simulink model "offline_snac_SITL"  (R2024a)
settings: Solver=FixedStepDiscrete  StartTime=0.0  StopTime=50  FixedStep=0.001  RelTol=1e-3  EnableMultiTasking=on
undefined symbols (not defined in the file or in its folder): DiscIntNeverNeededParam
libraries: simulink x6, px4uORBlib x3, sharedtransform x1, px4lib x1
settings Model: ExtModeTrigDuration=10  Creator=re606359  LastModifiedBy=engelhardt
settings SolverCC: PositivePriorityOrder=on
settings OptimizationCC: EnhancedBackFolding=on  PassReuseOutputArgsAs=Individual arguments  ZeroExternalMemoryAtStartup=off  ZeroInternalMemoryAtStartup=off  MaxStackSize=64  OptimizeBlockOrder=speed  DifferentSizesBufferReuse=on  OptimizationCustomize=off  EfficientTunableParamExpr=on
settings DebuggingCC: ParameterTunabilityLossMsg=error
settings HardwareCC: ProdBitPerPointer=32  ProdBitPerSizeT=32  ProdBitPerPtrDiffT=32  ProdLargestAtomicInteger=Long  ProdLargestAtomicFloat=Double  ProdWordSize=32  ProdLongLongMode=on  ProdHWDeviceType=ARM Compatible->ARM Cortex
settings SFSimCC: MATLABDynamicMemAlloc=off  SimTargetLang=C++
settings RTWCC: Description=Embedded Coder  SystemTargetFile=ert.tlc  HardwareBoard=PX4 Host Target  TLCOptions="-aInlineSetEventsForThisBaseRateFcn=TLC_FALSE -aSuppressMultiTaskScheduler=TLC_FALSE  -aRateBasedStepFcn=0"  TemplateMakefile=ert_default_tmf  Toolchain=GNU Tools for PX4 Autopilots  PortableWordSizes=on  TargetLang=C++  GPUComputeCapability=3.5
settings CodeAppCC: ForceParamTrailComments=on  IgnoreCustomStorageClasses=off  OperatorAnnotations=on  SimulinkDataObjDesc=on  SFDataObjDesc=on  InsertBlockDesc=on
settings ERTTargetCC: SupportContinuousTime=on  ExtModeTransport=2  ExtModeStaticAlloc=on  ExtModeMexFile=ext_xcp  ExtModeIntrfLevel=Level2 - Open

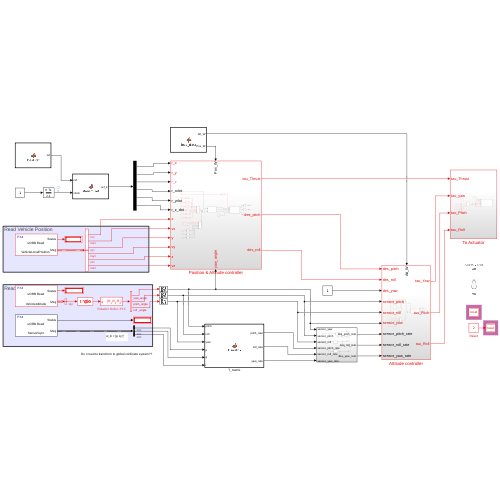
[thumbnail: Simulink's stored preview of the top-level diagram]
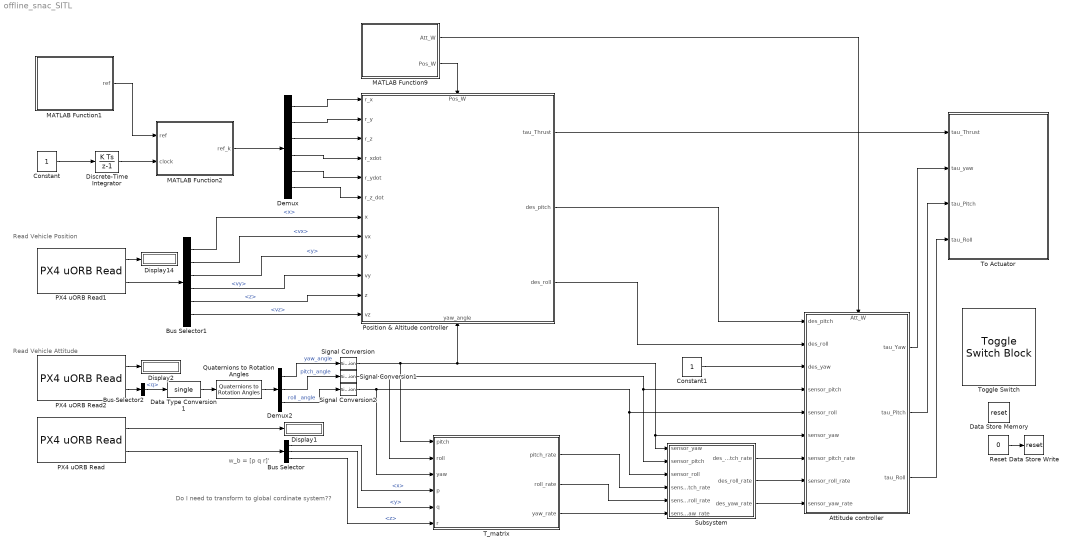
== system offline_snac_SITL ==
  note: w_b = [p q r]'
  note: Do I need to transform to global cordinate system??
  note: Read Vehicle Position
  note: Read Vehicle Attitude
  Attitude controller : Subsystem
      settings: PortSchema="{\"entries\":[{\"content\":{\"sides\":[{\"content\":{\"connectorIds\":[\"In1\",\"In2\",\"In3\",\"In4\",\"In5\",\"In6\",\"In7\",\"In8\",\"In9\"]},\"type\":\"ConnectorPlacement.EquallySpacedRectSide\",\"uuid\":\"fae962e8-eaa0-4300-aebb-2542e8dc0b9d\"},{\"content\":{\"connectorIds\":[\"Out1\",\"Out2\",\"Out3\"],\"side\":\"RIGHT\"},\"type\":\"ConnectorPlacement.EquallySpacedRectSide\",\"uuid\":\"2ab64516-4178-4987-b105-e2b60ebc653b\"},{\"content\":{\"connectorIds\":[\"In10\"],\"side\":\"TOP\"},\"type\":\"ConnectorPlacement.EquallySpacedRectSide\",\"uuid\":\"8c218eee-bea7-4b7a-ab96-9bd58138bc2f\"},{\"content\":{\"side\":\"BOTTOM\"},\"type\":\"ConnectorPlacement.EquallySpacedRectSide\",\"uuid\":\"12c5faa8-5812-413f-bdcf-aa5ffbd59e54\"}]},\"type\":\"ConnectorPlacement.EquallySpacedConnector\",\"uuid\":\"49b20a1e-3c6c-4df6-a9b5-cb8878061c64\"}],\"packageUris\":[\"http://schema.mathworks.com/mf0/Connector/R2020b\"],\"version\":\"1.0\"}"
  Bus Selector : BusSelector  OutputSignals=x,y,z
  Bus Selector1 : BusSelector  OutputSignals=x,vx,y,vy,z,vz
  Bus Selector2 : BusSelector  OutputSignals=q
  Constant : Constant  OutDataTypeStr=single
  Constant1 : Constant  OutDataTypeStr=single
  Data Store Write : DataStoreWrite  DataStoreName=reset  IndexOptions=Index vector (dialog)  Indices=1  OutputSizes=1
  Data Store Memory : DataStoreMemory  DataStoreName=reset  ReadBeforeWriteMsg=warning  WriteAfterWriteMsg=warning  WriteAfterReadMsg=warning  ShowAdditionalParam=off  OutDataTypeStr=boolean
  Data Type Conversion1 : DataTypeConversion  OutDataTypeStr=single  SaturateOnIntegerOverflow=off  RndMeth=Floor
  Demux : Demux  Outputs=6
  Demux2 : Demux  Outputs=3
  Discrete-Time Integrator : DiscreteIntegrator  SampleTime=-1  ICPrevOutput=DiscIntNeverNeededParam  ICPrevScaledInput=DiscIntNeverNeededParam
  Display1 : Display
  Display14 : Display
  Display2 : Display
  MATLAB Function1 : MATLAB Function  TreatAsAtomicUnit=on
  MATLAB Function2 : MATLAB Function  TreatAsAtomicUnit=on
  MATLAB Function9 : MATLAB Function  TreatAsAtomicUnit=on
  PX4 uORB Read : px4uORBlib/PX4 uORB Read  uORBTopic=SensorGyro  selectInstance=SensorGyro  SampleTime=-1  BlockingMode=off  BlockTimeout=1e-3
  PX4 uORB Read1 : px4uORBlib/PX4 uORB Read  uORBTopic=VehicleLocalPosition  selectInstance=vehicle_local_position  SampleTime=-1  BlockingMode=off  BlockTimeout=1e-3
  PX4 uORB Read2 : px4uORBlib/PX4 uORB Read  uORBTopic=VehicleAttitude  selectInstance=vehicle_attitude  SampleTime=-1  BlockingMode=off  BlockTimeout=1e-3
  Position & Altitude controller : Subsystem
      settings: PortSchema="{\"entries\":[{\"content\":{\"sides\":[{\"content\":{\"connectorIds\":[\"In1\",\"In2\",\"In3\",\"In4\",\"In5\",\"In6\",\"In7\",\"In8\",\"In9\",\"In10\",\"In11\",\"In12\"]},\"type\":\"ConnectorPlacement.EquallySpacedRectSide\",\"uuid\":\"96eb1e1d-33f8-43b2-aca1-3a2ea17c97d3\"},{\"content\":{\"connectorIds\":[\"Out1\",\"Out2\",\"Out3\"],\"side\":\"RIGHT\"},\"type\":\"ConnectorPlacement.EquallySpacedRectSide\",\"uuid\":\"68c63f59-0b7f-4dee-beff-edcde1fd911b\"},{\"content\":{\"connectorIds\":[\"In13\"],\"side\":\"TOP\"},\"type\":\"ConnectorPlacement.EquallySpacedRectSide\",\"uuid\":\"695c40b8-e625-4f49-aae8-ed972e1604cc\"},{\"content\":{\"connectorIds\":[\"In14\"],\"side\":\"BOTTOM\"},\"type\":\"ConnectorPlacement.EquallySpacedRectSide\",\"uuid\":\"eed3d45c-6018-4bc3-85c5-6c8aa0ab95cc\"}]},\"type\":\"ConnectorPlacement.EquallySpacedConnector\",\"uuid\":\"b4b28bb8-7674-4138-b24e-55baa1b4cc5c\"}],\"packageUris\":[\"http://schema.mathworks.com/mf0/Connector/R2020b\"],\"version\":\"1.0\"}"
  Quaternions to Rotation Angles : sharedtransform/Quaternions to Rotation Angles  rotationOrder=ZYX  aMode=aMode
  Reset : Constant  Value=0  OutDataTypeStr=boolean  SampleTime=-1
      settings: OpenFcn=|
      | if strcmp('0',get_param(gcb, 'Value'))                        set_param(gcb, 'Value', '1');
      | else
      |             set_param(gcb, 'Value', '0');
      | end
  Signal Conversion : SignalConversion  OverrideOpt=off
  Signal Conversion1 : SignalConversion  OverrideOpt=off
  Signal Conversion2 : SignalConversion  OverrideOpt=off
  Subsystem : Subsystem
  T_matrix : MATLAB Function  TreatAsAtomicUnit=on
  To Actuator : Subsystem
  Toggle Switch : ToggleSwitchBlock
      settings: Values={{'Off', 'On'}, [0 1]}
  wires:
  Bus Selector1/5 -> Position & Altitude controller/11(z)  "<z>"
  Demux2/1 -> Signal Conversion/1  "yaw_angle"
  PX4 uORB Read2/2 -> Bus Selector2/1
  Position & Altitude controller/1(tau_Thrust) -> To Actuator/1(tau_Thrust)
  Attitude controller/2(tau_Pitch) -> To Actuator/3(tau_Pitch)
  Demux2/3 -> Signal Conversion2/1  "roll _angle"
  Position & Altitude controller/3(des_roll) -> Attitude controller/2(des_roll)
  Signal Conversion/1 -> T_matrix/1(pitch), Attitude controller/6(sensor_yaw), Subsystem/1(sensor_yaw), Position & Altitude controller/14(yaw_angle)
  Bus Selector1/3 -> Position & Altitude controller/9(y)  "<y>"
  Attitude controller/1(tau_Yaw) -> To Actuator/2(tau_yaw)
  Quaternions to Rotation Angles/1 -> Demux2/1
  Bus Selector1/6 -> Position & Altitude controller/12(vz)  "<vz>"
  PX4 uORB Read2/1 -> Display2/1
  Position & Altitude controller/2(des_pitch) -> Attitude controller/1(des_pitch)
  Attitude controller/3(tau_Roll) -> To Actuator/4(tau_Roll)
  Demux2/2 -> Signal Conversion1/1  "pitch_angle"
  PX4 uORB Read1/1 -> Display14/1
  PX4 uORB Read1/2 -> Bus Selector1/1
  Signal Conversion1/1 -> T_matrix/2(roll), Subsystem/2(sensor_pitch), Attitude controller/4(sensor_pitch)
  Signal Conversion2/1 -> T_matrix/3(yaw), Subsystem/3(sensor_roll), Attitude controller/5("sensor_roll ")
  Bus Selector1/1 -> Position & Altitude controller/7(x)  "<x>"
  Bus Selector1/4 -> Position & Altitude controller/10(vy)  "<vy>"
  Bus Selector1/2 -> Position & Altitude controller/8(vx)  "<vx>"
  Reset/1 -> Data Store Write/1
  Bus Selector2/1 -> Data Type Conversion1/1  "<q>"
  Data Type Conversion1/1 -> Quaternions to Rotation Angles/1
  MATLAB Function9/2(Pos_W) -> Position & Altitude controller/13(Pos_W)
  MATLAB Function9/1(Att_W) -> Attitude controller/10(Att_W)
  PX4 uORB Read/1 -> Display1/1
  PX4 uORB Read/2 -> Bus Selector/1
  T_matrix/1(pitch_rate) -> Subsystem/4(sensor_pitch_rate)
  T_matrix/3(yaw_rate) -> Subsystem/6(sensor_yaw_rate)
  Bus Selector/1 -> T_matrix/4(p)  "<x>"
  Bus Selector/2 -> T_matrix/5(q)  "<y>"
  Bus Selector/3 -> T_matrix/6(r)  "<z>"
  T_matrix/2(roll_rate) -> Subsystem/5(sensor_roll_rate)
  MATLAB Function1/1(ref) -> MATLAB Function2/1(ref)
  Discrete-Time Integrator/1 -> MATLAB Function2/2(clock)
  Constant/1 -> Discrete-Time Integrator/1
  MATLAB Function2/1(ref_k) -> Demux/1
  Demux/1 -> Position & Altitude controller/1(r_x)
  Demux/2 -> Position & Altitude controller/2(r_y)
  Demux/3 -> Position & Altitude controller/3(r_z)
  Demux/4 -> Position & Altitude controller/4(r_xdot)
  Demux/5 -> Position & Altitude controller/5(r_ydot)
  Demux/6 -> Position & Altitude controller/6(r_z_dot)
  Subsystem/1(des_pitch_rate) -> Attitude controller/7(sensor_pitch_rate)
  Subsystem/2(des_roll_rate) -> Attitude controller/8(sensor_roll_rate)
  Subsystem/3(des_yaw_rate) -> Attitude controller/9(sensor_yaw_rate)
  Constant1/1 -> Attitude controller/3(des_yaw)

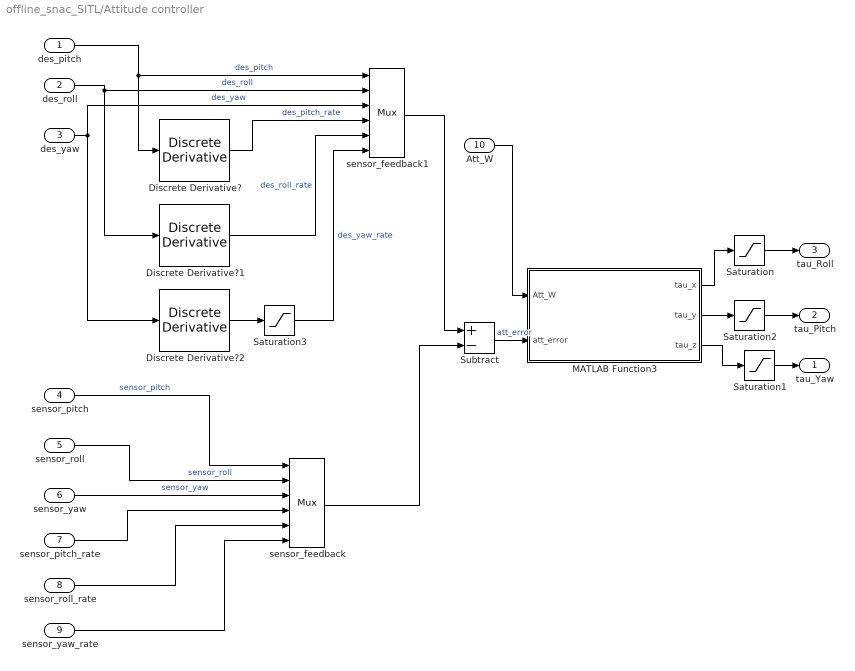
== system offline_snac_SITL/Attitude controller ==
  des_pitch : Inport  OutDataTypeStr=single
  des_roll : Inport  Port=2  OutDataTypeStr=single
  des_yaw : Inport  Port=3  OutDataTypeStr=single
  sensor_pitch : Inport  Port=4
  "sensor_roll " : Inport  Port=5
  sensor_yaw : Inport  Port=6
  sensor_pitch_rate : Inport  Port=7
  sensor_roll_rate : Inport  Port=8
  sensor_yaw_rate : Inport  Port=9
  Att_W : Inport  Port=10
  Discrete Derivative? : simulink/Discrete/Discrete Derivative  gainval=1.0  ICPrevScaledInput=0.0  OutMin=[]  OutMax=[]  OutDataTypeStr=single  OutputDataTypeScalingMode=single  OutDataType=fixdt(1, 16)  OutScaling=2^-10  DoSatur=off
  Discrete Derivative?1 : simulink/Discrete/Discrete Derivative  gainval=1.0  ICPrevScaledInput=0.0  OutMin=[]  OutMax=[]  OutDataTypeStr=single  OutputDataTypeScalingMode=single  OutDataType=fixdt(1, 16)  OutScaling=2^-10  DoSatur=off
  Discrete Derivative?2 : simulink/Discrete/Discrete Derivative  gainval=1.0  ICPrevScaledInput=0.0  OutMin=[]  OutMax=[]  OutDataTypeStr=single  OutputDataTypeScalingMode=single  OutDataType=fixdt(1, 16)  OutScaling=2^-10  DoSatur=off
  MATLAB Function3 : MATLAB Function  TreatAsAtomicUnit=on
  Saturation : Saturate  UpperLimit=8  LowerLimit=-8
  Saturation1 : Saturate  UpperLimit=3  LowerLimit=-3
  Saturation2 : Saturate  UpperLimit=8  LowerLimit=-8
  Saturation3 : Saturate  UpperLimit=1  LowerLimit=-1
  Subtract : Sum  Inputs=+-
  sensor_feedback : Mux  Inputs=6
  sensor_feedback1 : Mux  Inputs=6
  tau_Yaw : Outport
  tau_Pitch : Outport  Port=2
  tau_Roll : Outport  Port=3
  wires:
  sensor_pitch/1 -> sensor_feedback/1  "sensor_pitch"
  "sensor_roll "/1 -> sensor_feedback/2  "sensor_roll"
  sensor_yaw/1 -> sensor_feedback/3  "sensor_yaw"
  sensor_pitch_rate/1 -> sensor_feedback/4
  sensor_roll_rate/1 -> sensor_feedback/5
  sensor_yaw_rate/1 -> sensor_feedback/6
  sensor_feedback/1 -> Subtract/2
  Att_W/1 -> MATLAB Function3/1(Att_W)
  Subtract/1 -> MATLAB Function3/2(att_error)  "att_error"
  des_pitch/1 -> Discrete Derivative?/1, sensor_feedback1/1  "des_pitch"
  des_roll/1 -> Discrete Derivative?1/1, sensor_feedback1/2  "des_roll"
  des_yaw/1 -> Discrete Derivative?2/1, sensor_feedback1/3  "des_yaw"
  Saturation3/1 -> sensor_feedback1/6  "des_yaw_rate"
  Discrete Derivative?1/1 -> sensor_feedback1/5  "des_roll_rate"
  Discrete Derivative?/1 -> sensor_feedback1/4  "des_pitch_rate"
  sensor_feedback1/1 -> Subtract/1
  MATLAB Function3/1(tau_x) -> Saturation/1
  Saturation/1 -> tau_Roll/1
  Saturation2/1 -> tau_Pitch/1
  MATLAB Function3/2(tau_y) -> Saturation2/1
  Saturation1/1 -> tau_Yaw/1
  MATLAB Function3/3(tau_z) -> Saturation1/1
  Discrete Derivative?2/1 -> Saturation3/1

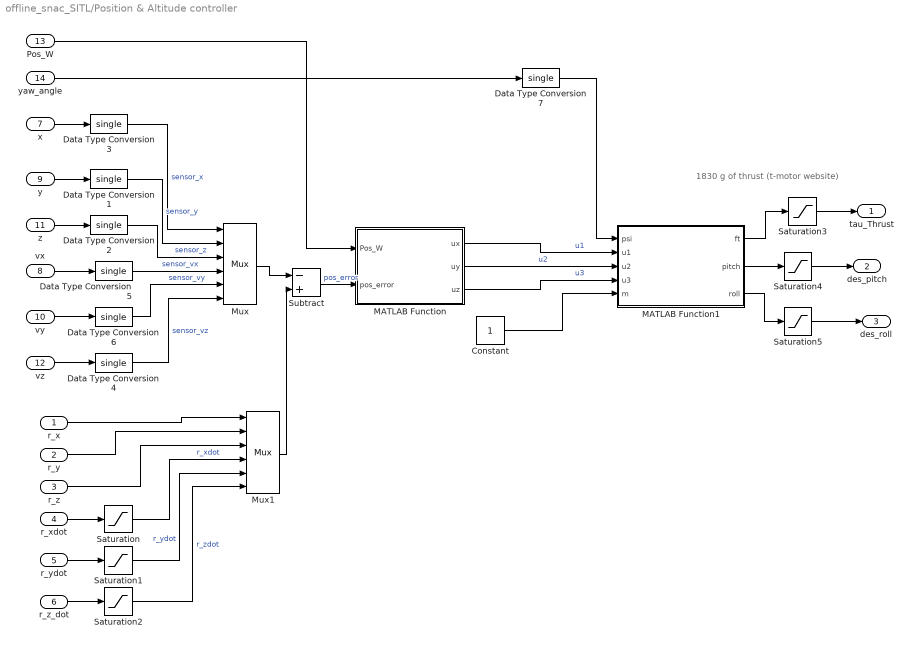
== system offline_snac_SITL/Position & Altitude controller ==
  note: 1830 g of thrust (t-motor website)
  r_x : Inport
  r_y : Inport  Port=2
  r_z : Inport  Port=3
  r_xdot : Inport  Port=4
  r_ydot : Inport  Port=5
  r_z_dot : Inport  Port=6
  x : Inport  Port=7
  vx : Inport  Port=8
  y : Inport  Port=9
  vy : Inport  Port=10
  z : Inport  Port=11
  vz : Inport  Port=12
  Pos_W : Inport  Port=13
  yaw_angle : Inport  Port=14
  Constant : Constant  OutDataTypeStr=single
  Data Type Conversion{1..7} (7 alike) : DataTypeConversion  OutDataTypeStr=single  SaturateOnIntegerOverflow=off  RndMeth=Floor
  MATLAB Function : MATLAB Function  TreatAsAtomicUnit=on
  MATLAB Function1 : MATLAB Function  TreatAsAtomicUnit=on
  Mux : Mux  Inputs=6
  Mux1 : Mux  Inputs=6
  Saturation : Saturate  UpperLimit=15  LowerLimit=-15
  Saturation1 : Saturate  UpperLimit=15  LowerLimit=-15
  Saturation2 : Saturate  UpperLimit=15  LowerLimit=-15
  Saturation3 : Saturate  UpperLimit=72  LowerLimit=0
  Saturation4 : Saturate  UpperLimit=.79  LowerLimit=-.79
  Saturation5 : Saturate  UpperLimit=.79  LowerLimit=-.79
  Subtract : Sum  Inputs=-+
  tau_Thrust : Outport  OutDataTypeStr=single
  des_pitch : Outport  Port=2
  des_roll : Outport  Port=3
  wires:
  z/1 -> Data Type Conversion2/1
  x/1 -> Data Type Conversion3/1
  y/1 -> Data Type Conversion1/1
  vz/1 -> Data Type Conversion4/1
  vx/1 -> Data Type Conversion5/1
  vy/1 -> Data Type Conversion6/1
  Pos_W/1 -> MATLAB Function/1(Pos_W)
  Data Type Conversion3/1 -> Mux/1  "sensor_x"
  Data Type Conversion1/1 -> Mux/2  "sensor_y"
  Data Type Conversion2/1 -> Mux/3  "sensor_z"
  Data Type Conversion5/1 -> Mux/4  "sensor_vx"
  Data Type Conversion6/1 -> Mux/5  "sensor_vy"
  Data Type Conversion4/1 -> Mux/6  "sensor_vz"
  Mux/1 -> Subtract/1
  Mux1/1 -> Subtract/2
  r_x/1 -> Mux1/1
  r_y/1 -> Mux1/2
  r_z/1 -> Mux1/3
  Subtract/1 -> MATLAB Function/2(pos_error)  "pos_error"
  Constant/1 -> MATLAB Function1/5(m)
  MATLAB Function/1(ux) -> MATLAB Function1/2(u1)  "u1"
  yaw_angle/1 -> Data Type Conversion7/1
  MATLAB Function/2(uy) -> MATLAB Function1/3(u2)  "u2"
  MATLAB Function/3(uz) -> MATLAB Function1/4(u3)  "u3"
  Data Type Conversion7/1 -> MATLAB Function1/1(psi)
  r_ydot/1 -> Saturation1/1
  r_z_dot/1 -> Saturation2/1
  r_xdot/1 -> Saturation/1
  Saturation/1 -> Mux1/4  "r_xdot"
  Saturation1/1 -> Mux1/5  "r_ydot"
  Saturation2/1 -> Mux1/6  "r_zdot"
  Saturation3/1 -> tau_Thrust/1
  MATLAB Function1/1(ft) -> Saturation3/1
  MATLAB Function1/2(pitch) -> Saturation4/1
  Saturation4/1 -> des_pitch/1
  Saturation5/1 -> des_roll/1
  MATLAB Function1/3(roll) -> Saturation5/1

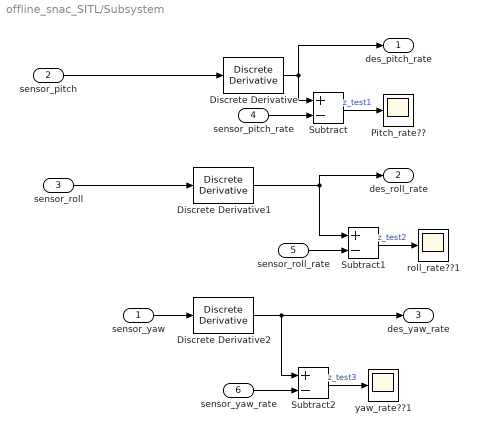
== system offline_snac_SITL/Subsystem ==
  sensor_yaw : Inport
  sensor_pitch : Inport  Port=2
  sensor_roll : Inport  Port=3
  sensor_pitch_rate : Inport  Port=4
  sensor_roll_rate : Inport  Port=5
  sensor_yaw_rate : Inport  Port=6
  Discrete Derivative : simulink/Discrete/Discrete Derivative  gainval=1.0  ICPrevScaledInput=0.0  OutMin=[]  OutMax=[]  OutDataTypeStr=single  OutputDataTypeScalingMode=single  OutDataType=fixdt(1, 16)  OutScaling=2^-10  DoSatur=off
  Discrete Derivative1 : simulink/Discrete/Discrete Derivative  gainval=1.0  ICPrevScaledInput=0.0  OutMin=[]  OutMax=[]  OutDataTypeStr=single  OutputDataTypeScalingMode=single  OutDataType=fixdt(1, 16)  OutScaling=2^-10  DoSatur=off
  Discrete Derivative2 : simulink/Discrete/Discrete Derivative  gainval=1.0  ICPrevScaledInput=0.0  OutMin=[]  OutMax=[]  OutDataTypeStr=single  OutputDataTypeScalingMode=single  OutDataType=fixdt(1, 16)  OutScaling=2^-10  DoSatur=off
  Pitch_rate?? : Scope
  Subtract : Sum  Inputs=+-
  Subtract1 : Sum  Inputs=+-
  Subtract2 : Sum  Inputs=+-
  roll_rate??1 : Scope
  yaw_rate??1 : Scope
  des_pitch_rate : Outport
  des_roll_rate : Outport  Port=2
  des_yaw_rate : Outport  Port=3
  wires:
  Subtract/1 -> Pitch_rate??/1  "z_test1"
  sensor_yaw_rate/1 -> Subtract2/2
  Discrete Derivative2/1 -> Subtract2/1, des_yaw_rate/1
  Subtract1/1 -> roll_rate??1/1  "z_test2"
  Discrete Derivative1/1 -> Subtract1/1, des_roll_rate/1
  sensor_roll/1 -> Discrete Derivative1/1
  Discrete Derivative/1 -> Subtract/1, des_pitch_rate/1
  sensor_pitch/1 -> Discrete Derivative/1
  sensor_yaw/1 -> Discrete Derivative2/1
  sensor_roll_rate/1 -> Subtract1/2
  Subtract2/1 -> yaw_rate??1/1  "z_test3"
  sensor_pitch_rate/1 -> Subtract/2

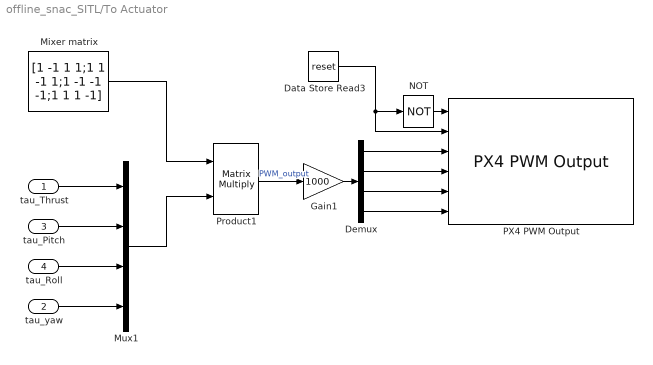
== system offline_snac_SITL/To Actuator ==
  tau_Thrust : Inport
  tau_yaw : Inport  Port=2
  tau_Pitch : Inport  Port=3
  tau_Roll : Inport  Port=4
  Data Store Read3 : DataStoreRead  DataStoreName=reset  IndexOptions=Index vector (dialog)  Indices=1  OutputSizes=1
  Demux : Demux
  Gain1 : Gain  Gain=1000  OutDataTypeStr=uint16
  Mixer matrix : Constant  Value=[1 -1 1 1;1 1 -1 1;1 -1 -1 -1;1 1 1 -1]  OutDataTypeStr=Inherit: Inherit via back propagation
  Mux1 : Mux
  NOT : Logic  Operator=NOT  IconShape=distinctive  AllPortsSameDT=off  OutDataTypeStr=boolean
  PX4 PWM Output : px4lib/PX4 PWM Output  pwmDevice=Main  pwmChannel1_=on  pwmChannel2_=on  pwmChannel3_=on  pwmChannel4_=on  pwmChannel5_=off  pwmChannel6_=off  pwmChannel7_=off  pwmChannel8_=off
  Product1 : Product  Multiplication=Matrix(*)  RndMeth=Zero
  wires:
  tau_Pitch/1 -> Mux1/2
  Mixer matrix/1 -> Product1/1
  tau_yaw/1 -> Mux1/4
  Mux1/1 -> Product1/2
  tau_Roll/1 -> Mux1/3
  tau_Thrust/1 -> Mux1/1
  Demux/1 -> PX4 PWM Output/3
  Demux/2 -> PX4 PWM Output/4
  Demux/3 -> PX4 PWM Output/5
  Demux/4 -> PX4 PWM Output/6
  Product1/1 -> Gain1/1  "PWM_output"
  Gain1/1 -> Demux/1
  NOT/1 -> PX4 PWM Output/1
  Data Store Read3/1 -> PX4 PWM Output/2, NOT/1

== matlab function offline_snac_SITL/MATLAB Function1 ==
  data: ref output
function ref = load_ref()

    data = coder.load('reference_SITL.mat', 'ref_states');    
    % Extract and convert the matrices to double
    ref = single(data.ref_states);
                


end

== matlab function offline_snac_SITL/MATLAB Function2 ==
  data: ref_k output; ref input; clock input
function ref_k = stream_ref(ref, clock)
    sample_time = 0.001;
    index = round(clock / sample_time) + 1; % Convert time to index
    index = min(index, size(ref, 2)); % Prevent index overflow
    ref_k = ref(:, index);

end

== matlab function offline_snac_SITL/Position & Altitude controller/MATLAB Function ==
  data: Pos_W input; pos_error input; ux output; uy output; uz output
function [ux, uy, uz] = position_control(Pos_W, pos_error)
        
        dt = single(0.001);
        Position_R = single(dt*diag([0.5e4,0.5e4,0.5e4]));
        Position_G = @(x) [0 0 0; 0 0 0; 0 0 0; -1 0 0; 0 -1 0; 0 0 -1] * dt;

        uxyz = -Position_R^-1 * Position_G( pos_error )' * Pos_W' * Basis_Func_84(pos_error );
        
        ux = single(zeros(1,1));
        uy = single(zeros(1,1));
        uz = single(zeros(1,1));
        
        ux = (uxyz(1));
        uy = (uxyz(2));
        uz = (uxyz(3));
        


end

function out = Basis_Func_84(x)
    % assert( isequal(size(x), [6, 1]),'Input must be a 6x1 matrix of real finite doubles.');
x1 = x(1);
x2 = x(2);
x3 = x(3);
x4 = x(4);
x5 = x(5);
x6 = x(6);

out = [1
    x1
    x2
    x3
    x4
    x5
    x6
    x1*x2
    x1*x3
    x1*x4
    x2*x3
    x1*x5
    x2*x4
    x1*x6
    x2*x5
    x3*x4
    x2*x6
    x3*x5
    x3*x6
    x4*x5
    x4*x6
    x5*x6
    x1*x2^2
    x1^2*x2
    x1*x3^2
    x1^2*x3
    x1*x4^2
    x2*x3^2
    x1^2*x4
    x2^2*x3
    x1*x5^2
    x2*x4^2
    x1^2*x5
    x2^2*x4
    x1*x6^2
    x2*x5^2
    x3*x4^2
    x1^2*x6
    x2^2*x5
    x3^2*x4
    x2*x6^2
    x3*x5^2
    x2^2*x6
    x3^2*x5
    x3*x6^2
    x4*x5^2
    x3^2*x6
    x4^2*x5
    x4*x6^2
    x4^2*x6
    x5*x6^2
    x5^2*x6
    x1^2
    x1^3
    x2^2
    x2^3
    x3^2
    x3^3
    x4^2
    x4^3
    x5^2
    x5^3
    x6^2
    x6^3
    x1*x2*x3
    x1*x2*x4
    x1*x2*x5
    x1*x3*x4
    x1*x2*x6
    x1*x3*x5
    x2*x3*x4
    x1*x3*x6
    x1*x4*x5
    x2*x3*x5
    x1*x4*x6
    x2*x3*x6
    x2*x4*x5
    x1*x5*x6
    x2*x4*x6
    x3*x4*x5
    x2*x5*x6
    x3*x4*x6
    x3*x5*x6
    x4*x5*x6
 ];
end

== matlab function offline_snac_SITL/Position & Altitude controller/MATLAB Function1 ==
  data: psi input; u1 input; u2 input; ft output; u3 input; m input; pitch output; roll output
function [ft, pitch, roll] = borna_sys_solve(psi, u1, u2, u3, m)

% make this more mem efficient later
    ft = single(zeros(1,1));
    pitch = single(zeros(1,1));
    roll = single(zeros(1,1));
    
    a = sin(psi);
    b = cos(psi);

    A = u1 / (u3);
    B = u2 / (u3);
    C = (a*A - b*B) / ( (a^2) + (b^2)) ;

    roll = single(atan( (B + b*C) / a ));
    pitch = single(atan( C * cos(roll) ));
    ft = ( m / (cos(pitch)*cos(roll)) ) * (-u3);



end

== matlab function offline_snac_SITL/MATLAB Function9 ==
  data: Att_W output; Pos_W output
function [Att_W, Pos_W] = load_data()

    data_thing = coder.load('trained_weights.mat', 'Position_W', 'Attitude_W');    
    % Extract and convert the matrices to double
    Pos_W = single(data_thing.Position_W);
    Att_W = single(data_thing.Attitude_W);
                


end

== matlab function offline_snac_SITL/Attitude controller/MATLAB Function3 ==
  data: Att_W input; att_error input; tau_x output; tau_y output; tau_z output
function [tau_x, tau_y, tau_z] = attitude_control(Att_W, att_error)
           
        dt = single(0.001);
        Ix = single(0.5); Iy = single(0.5); Iz = single(0.5);
        Attitude_R = dt*diag([0.5e4,0.5e4,0.5e4]);
        Attitude_G = [0 0 0; 0 0 0; 0 0 0; 1/Ix 0 0; 0 1/Iy 0; 0 0 1/Iz]*dt;


        torques = -Attitude_R^-1 * Attitude_G' * Att_W' * Basis_Func_84(att_error(:));
        tau_x = single(zeros(1,1));
        tau_y = single(zeros(1,1));
        tau_z = single(zeros(1,1));
        tau_x = (torques(1));
        tau_y = (torques(2));
        tau_z = (torques(3));

end

function out = Basis_Func_84(x)
    % assert( isequal(size(x), [6, 1]),'Input must be a 6x1 matrix of real finite doubles.');
x1 = x(1);
x2 = x(2);
x3 = x(3);
x4 = x(4);
x5 = x(5);
x6 = x(6);

out = [ 1
    x1
    x2
    x3
    x4
    x5
    x6
    x1*x2
    x1*x3
    x1*x4
    x2*x3
    x1*x5
    x2*x4
    x1*x6
    x2*x5
    x3*x4
    x2*x6
    x3*x5
    x3*x6
    x4*x5
    x4*x6
    x5*x6
    x1*x2^2
    x1^2*x2
    x1*x3^2
    x1^2*x3
    x1*x4^2
    x2*x3^2
    x1^2*x4
    x2^2*x3
    x1*x5^2
    x2*x4^2
    x1^2*x5
    x2^2*x4
    x1*x6^2
    x2*x5^2
    x3*x4^2
    x1^2*x6
    x2^2*x5
    x3^2*x4
    x2*x6^2
    x3*x5^2
    x2^2*x6
    x3^2*x5
    x3*x6^2
    x4*x5^2
    x3^2*x6
    x4^2*x5
    x4*x6^2
    x4^2*x6
    x5*x6^2
    x5^2*x6
    x1^2
    x1^3
    x2^2
    x2^3
    x3^2
    x3^3
    x4^2
    x4^3
    x5^2
    x5^3
    x6^2
    x6^3
    x1*x2*x3
    x1*x2*x4
    x1*x2*x5
    x1*x3*x4
    x1*x2*x6
    x1*x3*x5
    x2*x3*x4
    x1*x3*x6
    x1*x4*x5
    x2*x3*x5
    x1*x4*x6
    x2*x3*x6
    x2*x4*x5
    x1*x5*x6
    x2*x4*x6
    x3*x4*x5
    x2*x5*x6
    x3*x4*x6
    x3*x5*x6
    x4*x5*x6
 ];
end

== matlab function offline_snac_SITL/T_matrix ==
  data: pitch input; pitch_rate output; roll input; yaw input; p input; q input; r input; roll_rate output; yaw_rate output
function [pitch_rate, roll_rate, yaw_rate] = T_matrix(pitch, roll, yaw, p, q, r)

    w = [1,     sin(pitch)*tan(roll),       cos(pitch)*tan(roll)
        0,      cos(pitch),                 -sin(pitch)
        0,      sin(pitch)/cos(roll),       cos(pitch)/cos(roll)]*[p; q; r];
    pitch_rate= w(1);
    roll_rate= w(2);
    yaw_rate= w(3);

end
